simulink model "m20160728_2_3SecSnake3Drolling_2"  (R2021a)
settings: Solver=ode15s  StartTime=0.0  StopTime=15  FixedStep=1/1000  MaxStep=1  RelTol=1e-3  AbsTol=1e-3  EnableMultiTasking=on
undefined symbols (not defined in the file or in its folder): f20160722_2_3secNewCoGwcntcts_1_mex, f20160722_3_3sec_contactF_1_mex
libraries: simulink x2
settings Model: Creator=isuru  LastModifiedBy=Dimuthu
settings SolverCC: AutoScaleAbsTol=off  MaxOrder=1  ExtrapolationOrder=2  NumberNewtonIterations=2  ZeroCrossAlgorithm=Adaptive  AlgebraicLoopSolver=TrustRegion
settings DataIOCC: LimitDataPoints=on  SaveFormat=Array  ReturnWorkspaceOutputs=off
settings OptimizationCC: LifeSpan=inf
settings DebuggingCC: SolverPrmCheckMsg=warning  SFUnexpectedBacktrackingDiag=warning  SFNoUnconditionalDefaultTransitionDiag=warning  SFExecutionAtInitializationDiag=none  SFMachineParentedDataDiag=warning  ArithmeticOperatorsInVariantConditions=warning
settings ModelReferenceCC: EnableParallelModelReferenceBuilds=on  PropagateSignalLabelsOutOfModel=off
settings SFSimCC: SimUseLocalCustomCode=off  CustomCodeUndefinedFunction=UseInterfaceOnly
settings RTWCC: RTWUseLocalCustomCode=off  BuildConfiguration=Faster Runs
settings CodeAppCC: StateflowObjectComments=on
settings GRTTargetCC: TargetLangStandard=C89/C90 (ANSI)
settings ConfigComp: CovMetricSettings=dw  CovSaveCumulativeToWorkspaceVar=on  CovSaveSingleToWorkspaceVar=on  CovExternalEMLEnable=off  CovSFcnEnable=off

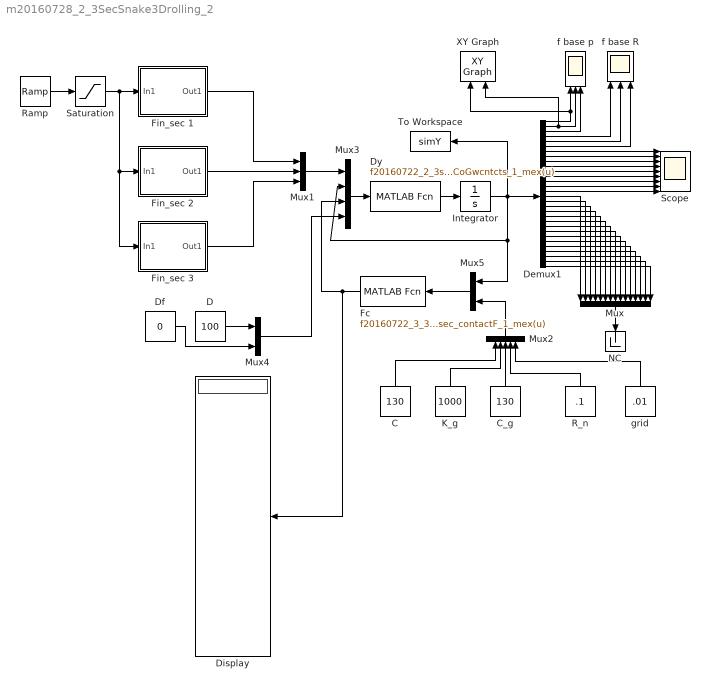
== system m20160728_2_3SecSnake3Drolling_2 ==
  C : Constant  Value=130
  C_g : Constant  Value=130
  D : Constant  Value=100
  Demux1 : Demux  Outputs=30
  Df : Constant  Value=0
  Display : Display
  Dy : MATLABFcn  MATLABFcn=f20160722_2_3secNewCoGwcntcts_1_mex(u)  OutputDimensions=30  OutputSignalType=real
  Fc : MATLABFcn  MATLABFcn=f20160722_3_3sec_contactF_1_mex(u)  OutputDimensions=15  OutputSignalType=real
  Fin_sec 1 : Subsystem
  Fin_sec 2 : Subsystem
  Fin_sec 3 : Subsystem
  Integrator : Integrator  InitialCondition=[0 0 0.6 pi/2+rand(1) 0 0 0 0 0 0 0 0 0 0 0 0 0 0 0 0 0 0 0 0 0 0 0 0 0 0]
  K_g : Constant  Value=1000
  Mux : Mux  Inputs=15
  Mux1 : Mux  Inputs=3
  Mux2 : Mux  Inputs=5
  Mux3 : Mux
  Mux4 : Mux  Inputs=2
  Mux5 : Mux  Inputs=2
  NC : Terminator
  R_n : Constant  Value=.1
  Ramp : simulink/Sources/Ramp  slope=1  start=.5  InitialOutput=0
  Saturation : Saturate  UpperLimit=1  LowerLimit=0
  Scope : Scope  NumInputPorts=9
  To Workspace : ToWorkspace  VariableName=simY  SaveFormat=Structure  SampleTime=1/30
  XY Graph : simulink/Sinks/XY Graph  xmin=-1  xmax=1  ymin=-1  ymax=1  st=-1
  f base R : Scope  NumInputPorts=3
  f base p : Scope  NumInputPorts=3
  grid : Constant  Value=.01
  wires:
  Dy/1 -> Integrator/1
  Integrator/1 -> Mux5/1, Mux3/2, Demux1/1, To Workspace/1
  Mux/1 -> NC/1
  Mux3/1 -> Dy/1
  Demux1/1 -> XY Graph/1, f base p/1
  Demux1/2 -> f base p/2, XY Graph/2
  Demux1/3 -> f base p/3
  Ramp/1 -> Saturation/1
  Demux1/9 -> Scope/3
  Demux1/8 -> Scope/2
  Demux1/7 -> Scope/1
  D/1 -> Mux4/1
  Df/1 -> Mux4/2
  Mux5/1 -> Fc/1
  Mux2/1 -> Mux5/2
  Mux4/1 -> Mux3/4
  Fc/1 -> Display/1, Mux3/3
  Demux1/4 -> f base R/1
  Demux1/5 -> f base R/2
  Demux1/6 -> f base R/3
  C_g/1 -> Mux2/3
  K_g/1 -> Mux2/2
  R_n/1 -> Mux2/4
  C/1 -> Mux2/1
  grid/1 -> Mux2/5
  Demux1/14 -> Scope/8
  Demux1/11 -> Scope/5
  Demux1/15 -> Scope/9
  Demux1/13 -> Scope/7
  Demux1/10 -> Scope/4
  Demux1/12 -> Scope/6
  Demux1/17 -> Mux/2
  Demux1/16 -> Mux/1
  Demux1/18 -> Mux/3
  Demux1/30 -> Mux/15
  Demux1/29 -> Mux/14
  Demux1/28 -> Mux/13
  Demux1/25 -> Mux/10
  Demux1/26 -> Mux/11
  Demux1/27 -> Mux/12
  Demux1/19 -> Mux/4
  Demux1/23 -> Mux/8
  Demux1/20 -> Mux/5
  Demux1/21 -> Mux/6
  Demux1/22 -> Mux/7
  Demux1/24 -> Mux/9
  Saturation/1 -> Fin_sec 3/1(In1), Fin_sec 2/1(In1), Fin_sec 1/1(In1)
  Fin_sec 2/1(Out1) -> Mux1/2
  Fin_sec 3/1(Out1) -> Mux1/3
  Fin_sec 1/1(Out1) -> Mux1/1
  Mux1/1 -> Mux3/1

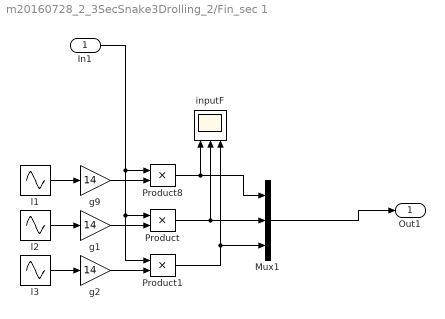
== system m20160728_2_3SecSnake3Drolling_2/Fin_sec 1 ==
  In1 : Inport
  Mux1 : Mux  Inputs=3
  Product : Product
  Product1 : Product
  Product8 : Product
  g1 : Gain  Gain=14
  g2 : Gain  Gain=14
  g9 : Gain  Gain=14
  inputF : Scope  NumInputPorts=3
  l1 : Sin  Bias=1  Frequency=2  SampleTime=0
  l2 : Sin  Bias=1  Frequency=2  Phase=2*pi/3  SampleTime=0
  l3 : Sin  Bias=1  Frequency=2  Phase=4*pi/3  SampleTime=0
  Out1 : Outport  VectorParamsAs1DForOutWhenUnconnected=off
  wires:
  Product/1 -> Mux1/2, inputF/2
  In1/1 -> Product8/1, Product/1, Product1/1
  Mux1/1 -> Out1/1
  l1/1 -> g9/1
  g1/1 -> Product/2
  g9/1 -> Product8/2
  g2/1 -> Product1/2
  Product1/1 -> Mux1/3, inputF/3
  Product8/1 -> Mux1/1, inputF/1
  l2/1 -> g1/1
  l3/1 -> g2/1

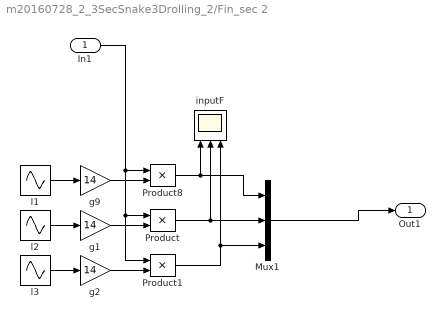
== system m20160728_2_3SecSnake3Drolling_2/Fin_sec 2 ==
  In1 : Inport
  Mux1 : Mux  Inputs=3
  Product : Product
  Product1 : Product
  Product8 : Product
  g1 : Gain  Gain=14
  g2 : Gain  Gain=14
  g9 : Gain  Gain=14
  inputF : Scope  NumInputPorts=3
  l1 : Sin  Bias=1  Frequency=2  Phase=0+pi/3  SampleTime=0
  l2 : Sin  Bias=1  Frequency=2  Phase=2*pi/3+pi/3  SampleTime=0
  l3 : Sin  Bias=1  Frequency=2  Phase=4*pi/3+pi/3  SampleTime=0
  Out1 : Outport  VectorParamsAs1DForOutWhenUnconnected=off
  wires:
  Product8/1 -> inputF/1, Mux1/1
  Product1/1 -> inputF/3, Mux1/3
  g2/1 -> Product1/2
  g9/1 -> Product8/2
  g1/1 -> Product/2
  l1/1 -> g9/1
  Mux1/1 -> Out1/1
  In1/1 -> Product1/1, Product/1, Product8/1
  Product/1 -> inputF/2, Mux1/2
  l2/1 -> g1/1
  l3/1 -> g2/1

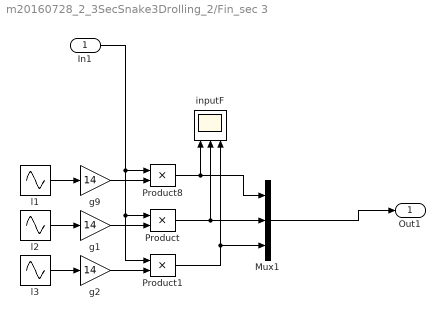
== system m20160728_2_3SecSnake3Drolling_2/Fin_sec 3 ==
  In1 : Inport
  Mux1 : Mux  Inputs=3
  Product : Product
  Product1 : Product
  Product8 : Product
  g1 : Gain  Gain=14
  g2 : Gain  Gain=14
  g9 : Gain  Gain=14
  inputF : Scope  NumInputPorts=3
  l1 : Sin  Bias=1  Frequency=2  Phase=0+2*pi/3  SampleTime=0
  l2 : Sin  Bias=1  Frequency=2  Phase=2*pi/3+2*pi/3  SampleTime=0
  l3 : Sin  Bias=1  Frequency=2  Phase=4*pi/3+2*pi/3  SampleTime=0
  Out1 : Outport  VectorParamsAs1DForOutWhenUnconnected=off
  wires:
  Product/1 -> Mux1/2, inputF/2
  In1/1 -> Product8/1, Product/1, Product1/1
  Mux1/1 -> Out1/1
  l1/1 -> g9/1
  g1/1 -> Product/2
  g9/1 -> Product8/2
  g2/1 -> Product1/2
  Product1/1 -> Mux1/3, inputF/3
  Product8/1 -> Mux1/1, inputF/1
  l2/1 -> g1/1
  l3/1 -> g2/1
